simulink model "linCartPendulumOF"  (R2020a)
settings: Solver=VariableStepAuto  StartTime=0.0  StopTime=10.0  RelTol=1e-3
values from neighbouring files (symbols this model uses):
  xinit = [0;0;0;0]    [setupModelParameters.m]
undefined symbols (not defined in the file or in its folder): A, Ahat, B, Bhat, C, Chat, Dhat, xhatinit
settings Model: Creator=jamess  LastModifiedBy=jamessaunderson
settings DataIOCC: ReturnWorkspaceOutputs=off
settings DebuggingCC: ArithmeticOperatorsInVariantConditions=warning
settings SFSimCC: SimUseLocalCustomCode=off  CustomCodeUndefinedFunction=UseInterfaceOnly
settings RTWCC: RTWUseLocalCustomCode=off
settings CodeAppCC: StateflowObjectComments=on

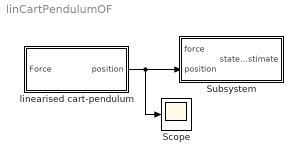
== system linCartPendulumOF ==
  Scope : Scope
  Subsystem : Subsystem
  linearised cart-pendulum : Subsystem
  wires:
  linearised cart-pendulum/1(position) -> Scope/1, Subsystem/2(position)

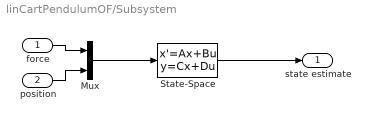
== system linCartPendulumOF/Subsystem ==
  force : Inport
  position : Inport  Port=2
  Mux : Mux  Inputs=2
  State-Space : StateSpace  A=Ahat  B=Bhat  C=Chat  D=Dhat  InitialCondition=xhatinit
  state estimate : Outport
  wires:
  State-Space/1 -> state estimate/1
  force/1 -> Mux/1
  position/1 -> Mux/2
  Mux/1 -> State-Space/1

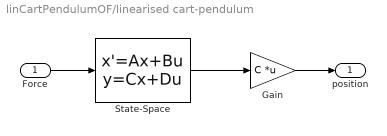
== system linCartPendulumOF/linearised cart-pendulum ==
  Force : Inport
  Gain : Gain  Gain=C  Multiplication=Matrix(K*u) (u vector)
  State-Space : StateSpace  A=A  B=B  C=eye(4)  D=zeros(4,1)  InitialCondition=xinit
  position : Outport
  wires:
  Force/1 -> State-Space/1
  State-Space/1 -> Gain/1
  Gain/1 -> position/1
